simulink library "MTBcontroller"  (R2014b)
settings: Solver=ode45  StartTime=0.0  StopTime=10.0  RelTol=1e-3
undefined symbols (not defined in the file or in its folder): ConfParam
libraries: ChangeFrame x1, ComputeNorm3D x1, DivisionVectorScalar x1, CrossProd x1
settings Model: Creator=Hp  LastModifiedBy=Hp

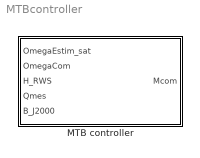
== system MTBcontroller ==
  MTB controller : Subsystem

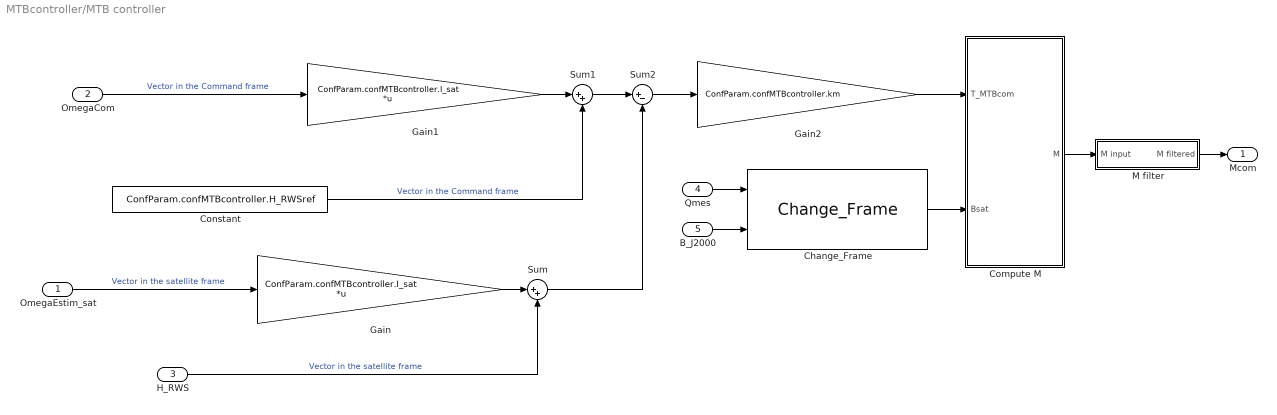
== system MTBcontroller/MTB controller ==
  OmegaEstim_sat : Inport
  OmegaCom : Inport  Port=2
  H_RWS : Inport  Port=3
  Qmes : Inport  Port=4
  B_J2000 : Inport  Port=5
  Change_Frame : ChangeFrame/Change_Frame
  Compute M : Subsystem
  Constant : Constant  Value=ConfParam.confMTBcontroller.H_RWSref
  Gain : Gain  Gain=ConfParam.confMTBcontroller.I_sat  Multiplication=Matrix(K*u)
  Gain1 : Gain  Gain=ConfParam.confMTBcontroller.I_sat  Multiplication=Matrix(K*u)
  Gain2 : Gain  Gain=ConfParam.confMTBcontroller.km
  M filter : Subsystem
  Sum : Sum  Inputs=|++
  Sum1 : Sum  Inputs=|++
  Sum2 : Sum  Inputs=|+-
  Mcom : Outport
  wires:
  Gain1/1 -> Sum1/1
  H_RWS/1 -> Sum/2  "Vector in the satellite frame"
  Sum1/1 -> Sum2/1
  OmegaEstim_sat/1 -> Gain/1  "Vector in the satellite frame"
  Sum2/1 -> Gain2/1
  Gain/1 -> Sum/1
  Constant/1 -> Sum1/2  "Vector in the Command frame"
  Sum/1 -> Sum2/2
  OmegaCom/1 -> Gain1/1  "Vector in the Command frame"
  Gain2/1 -> Compute M/1(T_MTBcom)
  B_J2000/1 -> Change_Frame/2
  Qmes/1 -> Change_Frame/1
  Change_Frame/1 -> Compute M/2(Bsat)
  Compute M/1(M) -> M filter/1(M input)
  M filter/1(M filtered) -> Mcom/1

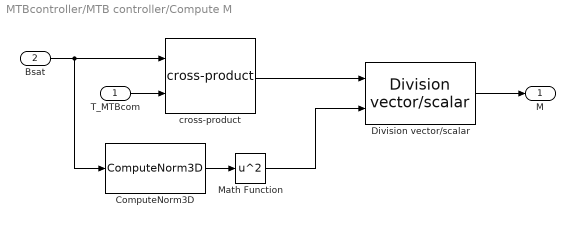
== system MTBcontroller/MTB controller/Compute M ==
  T_MTBcom : Inport
  Bsat : Inport  Port=2
  ComputeNorm3D : ComputeNorm3D/ComputeNorm3D
  Division vector/scalar : DivisionVectorScalar/Division vector//scalar
  Math Function : Math  Operator=square  SaturateOnIntegerOverflow=on
  cross-product : CrossProd/cross-product
  M : Outport
  wires:
  Division vector/scalar/1 -> M/1
  ComputeNorm3D/1 -> Math Function/1
  cross-product/1 -> Division vector/scalar/1
  T_MTBcom/1 -> cross-product/2
  Bsat/1 -> cross-product/1, ComputeNorm3D/1
  Math Function/1 -> Division vector/scalar/2

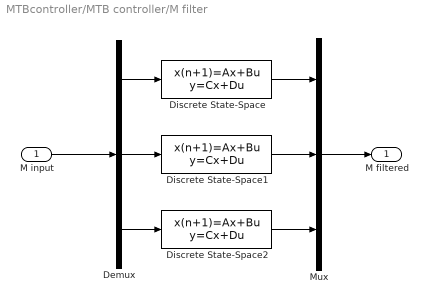
== system MTBcontroller/MTB controller/M filter ==
  M input : Inport
  Demux : Demux  Outputs=3
  Discrete State-Space : DiscreteStateSpace  A=ConfParam.confMTBcontroller.A  B=ConfParam.confMTBcontroller.B  C=ConfParam.confMTBcontroller.C  D=ConfParam.confMTBcontroller.D  X0=[0; 0]  SampleTime=1/ConfParam.confES.frequency
  Discrete State-Space1 : DiscreteStateSpace  A=ConfParam.confMTBcontroller.A  B=ConfParam.confMTBcontroller.B  C=ConfParam.confMTBcontroller.C  D=ConfParam.confMTBcontroller.D  X0=[0; 0]  SampleTime=1/ConfParam.confES.frequency
  Discrete State-Space2 : DiscreteStateSpace  A=ConfParam.confMTBcontroller.A  B=ConfParam.confMTBcontroller.B  C=ConfParam.confMTBcontroller.C  D=ConfParam.confMTBcontroller.D  X0=[0; 0]  SampleTime=1/ConfParam.confES.frequency
  Mux : Mux  Inputs=3
  M filtered : Outport
  wires:
  Demux/1 -> Discrete State-Space/1
  Mux/1 -> M filtered/1
  Demux/2 -> Discrete State-Space1/1
  Demux/3 -> Discrete State-Space2/1
  M input/1 -> Demux/1
  Discrete State-Space1/1 -> Mux/2
  Discrete State-Space/1 -> Mux/1
  Discrete State-Space2/1 -> Mux/3
